simulink model "Lev_project_control_no_obs"  (R2022b)
settings: Solver=VariableStepAuto  StartTime=0.0  StopTime=Tsim  FixedStep=0.01  RelTol=1e-3
values from neighbouring files (symbols this model uses):
  A = A-B*K0    [project.m]
  Ad = zeros(6,6)    [project.m]
  B = [0; -9.9453]    [project.m]
  C = [708.27 0]    [project.m]
  c = 1/(2*real(minimum_eig))    [project.m]
  D = 0    [project.m]
  G = diag([0 1 0 6 0 0])    [project.m]
  K = (R\B')*P    [project.m]
  x_0 = [0 0]'    [project.m]
  x_0_Leader = [0 2]'    [project.m]
libraries: matrix_library x6
settings Model: Creator=Matteo  LastModifiedBy=Soff

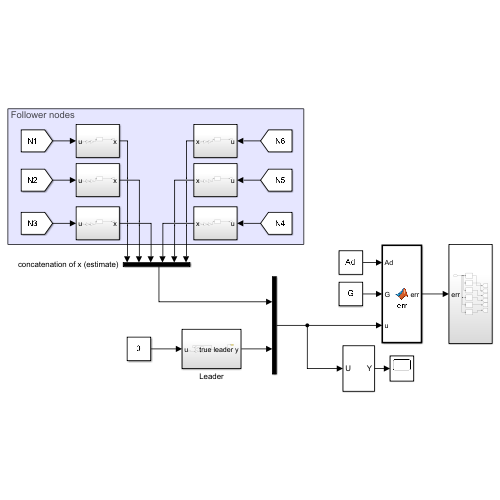
[thumbnail: Simulink's stored preview of the top-level diagram]
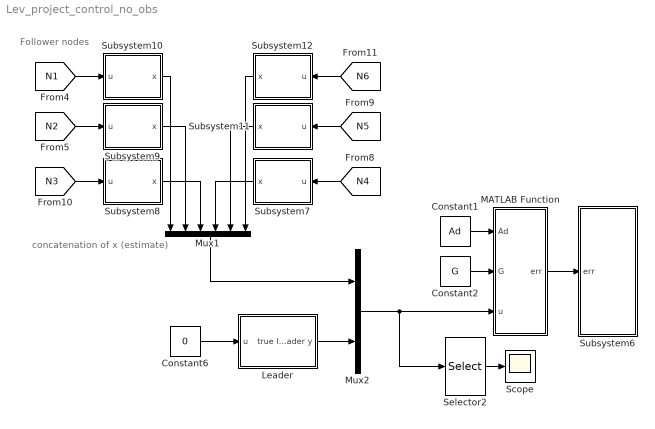
== system Lev_project_control_no_obs ==
  note: concatenation of x (estimate)
  note: Follower nodes
  Constant1 : Constant  Value=Ad
  Constant2 : Constant  Value=G
  Constant6 : Constant  Value=0
  Leader : Subsystem
  MATLAB Function : MATLAB Function  TreatAsAtomicUnit=on
  Mux1 : Mux  Inputs=6
  Mux2 : Mux  Inputs=2
  Scope : Scope
  Selector2 : Selector  InputPortWidth=14  IndexOptions=Index vector (dialog)  Indices=[1 3 5 7 9 11 13]  OutputSizes=1
  Subsystem10 : Subsystem
  Subsystem11 : Subsystem
  Subsystem12 : Subsystem
  Subsystem6 : Subsystem
  Subsystem7 : Subsystem
  Subsystem8 : Subsystem
  Subsystem9 : Subsystem
  wires:
  Selector2/1 -> Scope/1
  Constant1/1 -> MATLAB Function/1(Ad)
  Constant2/1 -> MATLAB Function/2(G)
  Mux2/1 -> Selector2/1, MATLAB Function/3(u)
  Leader/1(true leader y) -> Mux2/2
  MATLAB Function/1(err) -> Subsystem6/1(err)
  [N1] -> Subsystem10/1(u)
  [N4] -> Subsystem7/1(u)
  [N2] -> Subsystem9/1(u)
  [N3] -> Subsystem8/1(u)
  [N5] -> Subsystem11/1(u)
  [N6] -> Subsystem12/1(u)
  Subsystem10/1(x) -> Mux1/1
  Constant6/1 -> Leader/1(u)
  Subsystem9/1(x) -> Mux1/2
  Subsystem8/1(x) -> Mux1/3
  Subsystem7/1(x) -> Mux1/4
  Subsystem11/1(x) -> Mux1/5
  Subsystem12/1(x) -> Mux1/6
  Mux1/1 -> Mux2/1

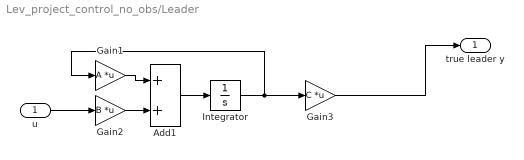
== system Lev_project_control_no_obs/Leader ==
  u : Inport
  Add1 : Sum
  Gain1 : Gain  Gain=A  Multiplication=Matrix(K*u)
  Gain2 : Gain  Gain=B  Multiplication=Matrix(K*u)
  Gain3 : Gain  Gain=C  Multiplication=Matrix(K*u)
  Integrator : Integrator  InitialCondition=x_0_Leader
  true leader y : Outport
  wires:
  Gain3/1 -> true leader y/1
  Gain1/1 -> Add1/1
  Gain2/1 -> Add1/2
  Add1/1 -> Integrator/1
  Integrator/1 -> Gain1/1, Gain3/1
  u/1 -> Gain2/1

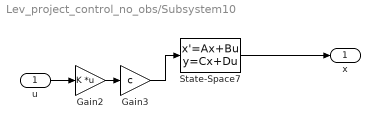
== system Lev_project_control_no_obs/Subsystem10 ==
  u : Inport
  Gain2 : Gain  Gain=K  Multiplication=Matrix(K*u)
  Gain3 : Gain  Gain=c
  State-Space7 : StateSpace  A=A  B=B  C=C  D=D  InitialCondition=x_0
  x : Outport
  wires:
  State-Space7/1 -> x/1
  u/1 -> Gain2/1
  Gain2/1 -> Gain3/1
  Gain3/1 -> State-Space7/1

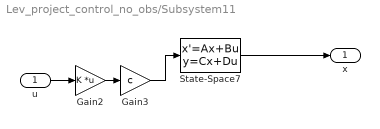
== system Lev_project_control_no_obs/Subsystem11 ==
  u : Inport
  Gain2 : Gain  Gain=K  Multiplication=Matrix(K*u)
  Gain3 : Gain  Gain=c
  State-Space7 : StateSpace  A=A  B=B  C=C  D=D  InitialCondition=x_0
  x : Outport
  wires:
  State-Space7/1 -> x/1
  Gain2/1 -> Gain3/1
  u/1 -> Gain2/1
  Gain3/1 -> State-Space7/1

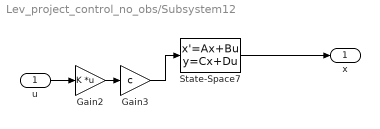
== system Lev_project_control_no_obs/Subsystem12 ==
  u : Inport
  Gain2 : Gain  Gain=K  Multiplication=Matrix(K*u)
  Gain3 : Gain  Gain=c
  State-Space7 : StateSpace  A=A  B=B  C=C  D=D  InitialCondition=x_0
  x : Outport
  wires:
  State-Space7/1 -> x/1
  Gain2/1 -> Gain3/1
  u/1 -> Gain2/1
  Gain3/1 -> State-Space7/1

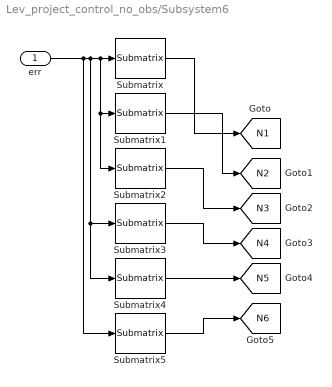
== system Lev_project_control_no_obs/Subsystem6 ==
  err : Inport
  Submatrix : matrix_library/Submatrix  RowSpan=All rows  RowStartMode=First  RowStartIndex=1  RowEndMode=Last  RowEndIndex=1  ColSpan=One column  ColStartMode=Index  ColStartIndex=1  ColEndMode=Last  ColEndIndex=1
  Submatrix1 : matrix_library/Submatrix  RowSpan=All rows  RowStartMode=First  RowStartIndex=1  RowEndMode=Last  RowEndIndex=1  ColSpan=One column  ColStartMode=Index  ColStartIndex=2  ColEndMode=Last  ColEndIndex=1
  Submatrix2 : matrix_library/Submatrix  RowSpan=All rows  RowStartMode=First  RowStartIndex=1  RowEndMode=Last  RowEndIndex=1  ColSpan=One column  ColStartMode=Index  ColStartIndex=3  ColEndMode=Last  ColEndIndex=1
  Submatrix3 : matrix_library/Submatrix  RowSpan=All rows  RowStartMode=First  RowStartIndex=1  RowEndMode=Last  RowEndIndex=1  ColSpan=One column  ColStartMode=Index  ColStartIndex=4  ColEndMode=Last  ColEndIndex=1
  Submatrix4 : matrix_library/Submatrix  RowSpan=All rows  RowStartMode=First  RowStartIndex=1  RowEndMode=Last  RowEndIndex=1  ColSpan=One column  ColStartMode=Index  ColStartIndex=5  ColEndMode=Last  ColEndIndex=1
  Submatrix5 : matrix_library/Submatrix  RowSpan=All rows  RowStartMode=First  RowStartIndex=1  RowEndMode=Last  RowEndIndex=1  ColSpan=One column  ColStartMode=Index  ColStartIndex=6  ColEndMode=Last  ColEndIndex=1
  tag scope: N1=global, N2=global, N3=global, N4=global, N5=global, N6=global
  wires:
  Submatrix4/1 -> [N5]
  Submatrix/1 -> [N1]
  Submatrix3/1 -> [N4]
  err/1 -> Submatrix5/1, Submatrix3/1, Submatrix4/1, Submatrix1/1, Submatrix2/1, Submatrix/1
  Submatrix5/1 -> [N6]
  Submatrix2/1 -> [N3]
  Submatrix1/1 -> [N2]

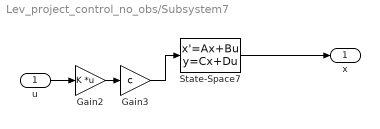
== system Lev_project_control_no_obs/Subsystem7 ==
  u : Inport
  Gain2 : Gain  Gain=K  Multiplication=Matrix(K*u)
  Gain3 : Gain  Gain=c
  State-Space7 : StateSpace  A=A  B=B  C=C  D=D  InitialCondition=x_0
  x : Outport
  wires:
  State-Space7/1 -> x/1
  Gain2/1 -> Gain3/1
  u/1 -> Gain2/1
  Gain3/1 -> State-Space7/1

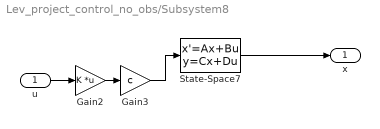
== system Lev_project_control_no_obs/Subsystem8 ==
  u : Inport
  Gain2 : Gain  Gain=K  Multiplication=Matrix(K*u)
  Gain3 : Gain  Gain=c
  State-Space7 : StateSpace  A=A  B=B  C=C  D=D  InitialCondition=x_0
  x : Outport
  wires:
  State-Space7/1 -> x/1
  Gain2/1 -> Gain3/1
  u/1 -> Gain2/1
  Gain3/1 -> State-Space7/1

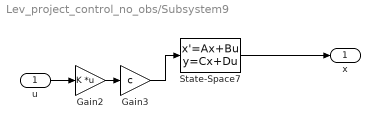
== system Lev_project_control_no_obs/Subsystem9 ==
  u : Inport
  Gain2 : Gain  Gain=K  Multiplication=Matrix(K*u)
  Gain3 : Gain  Gain=c
  State-Space7 : StateSpace  A=A  B=B  C=C  D=D  InitialCondition=x_0
  x : Outport
  wires:
  State-Space7/1 -> x/1
  Gain2/1 -> Gain3/1
  u/1 -> Gain2/1
  Gain3/1 -> State-Space7/1

== matlab function Lev_project_control_no_obs/MATLAB Function ==
  data: Ad input; G input; u input; err output
function err = err(Ad,G,u)

% state dimension (single node)
n = 2;

% number of follower nodes
m = 6;

x=zeros(n,m+1);

tmp = u';

for j = 1:m+1
    for i = 1:n
        x(i,j) = tmp(1);
        tmp = circshift(tmp,[0 -1]);
    end
%     x(:,j)
end

err = zeros(n,m);
for i = 1:m
%     err(:,i) = zeros(n,1);
    for x_component = 1:n
        %(x(x_component,m+1)-x(x_component,i))
        for j = 1:m
            err(x_component,i) = err(x_component,i) + Ad(i,j)*(x(x_component,j)-x(x_component,i));
        end
        
        err(x_component,i) = err(x_component,i) + G(i,i)*(x(x_component,m+1)-x(x_component,i));
    end
end
